simulink model "RL_Satellite_Model"  (R2024b)
settings: Solver=ode4  StartTime=0.0  StopTime=100  FixedStep=0.1  RelTol=1e-3
values from neighbouring files (symbols this model uses):
  debris1_vx = debris1_speed * cos(debris1_angle)    [agent_installation.m]    (also in resetFcn.m = 0.5*vx0 + debris1_speed * cos(dir1))
  debris1_vy = debris1_speed * sin(debris1_angle)    [agent_installation.m]    (also in resetFcn.m = 0.5*vy0 + debris1_speed * sin(dir1))
  debris1_vz = 0    [agent_installation.m]    (also in resetFcn.m = -(500 + rand*1000))
  debris2_vx = debris2_speed * cos(debris2_angle)    [agent_installation.m]    (also in resetFcn.m = 0.5*vx0 + debris2_speed * cos(dir2))
  debris2_vy = debris2_speed * sin(debris2_angle)    [agent_installation.m]    (also in resetFcn.m = 0.5*vy0 + debris2_speed * sin(dir2))
  debris2_vz = 0    [agent_installation.m]    (also in resetFcn.m = +(500 + rand*1000))
  debris3_vx = debris3_speed * cos(debris3_angle)    [agent_installation.m]    (also in resetFcn.m = 0.5*vx0 + debris3_speed * cos(dir3))
  debris3_vy = debris3_speed * sin(debris3_angle)    [agent_installation.m]    (also in resetFcn.m = 0.5*vy0 + debris3_speed * sin(dir3))
  debris3_vz = 0    [agent_installation.m]    (also in resetFcn.m = (rand - 0.5) * 300)
  vx0 = 0    [agent_installation.m]    (also in resetFcn.m = -sqrt(mu/r_target) * sin(sat_angle))
  vy0 = 7546    [agent_installation.m]    (also in resetFcn.m = sqrt(mu/r_target) * cos(sat_angle))
  vz0 = 0    [agent_installation.m]    (also in resetFcn.m)
  x0 = 7e6    (= 7000000)    [agent_installation.m]    (also in resetFcn.m = r_target * cos(sat_angle))
  y0 = 0    [agent_installation.m]    (also in resetFcn.m = r_target * sin(sat_angle))
  z0 = 0    [agent_installation.m]    (also in resetFcn.m = (rand - 0.5) * 2e4)
libraries: simulink x4, rllib x1, vrlib x1
settings Model: PacingRate=20  Creator=Emc  LastModifiedBy=Emc

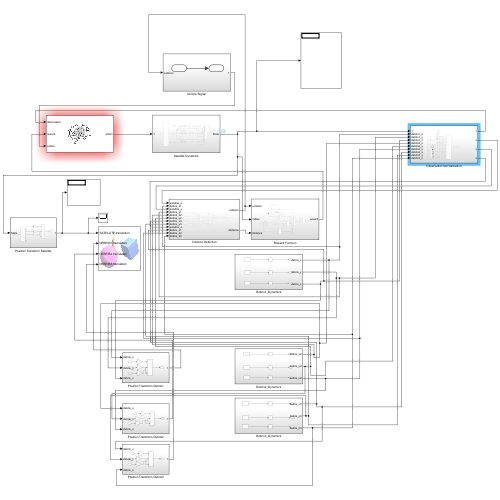
[thumbnail: Simulink's stored preview of the top-level diagram]
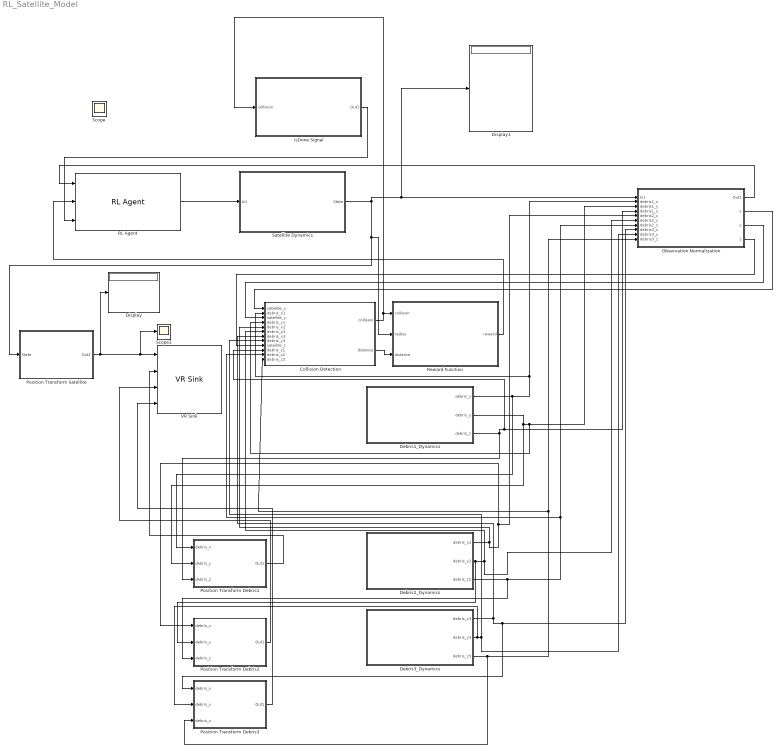
== system RL_Satellite_Model ==
  Collision Detection : Subsystem
  Debris1_Dynamics : Subsystem
  Debris2_Dynamics : Subsystem
  Debris3_Dynamics : Subsystem
  Display : Display
  Display1 : Display
  Observation Normalization : Subsystem
  Position Transform Debris1 : Subsystem
  Position Transform Debris2 : Subsystem
  Position Transform Debris3 : Subsystem
  Position Transform Satellite : Subsystem
  RL Agent : rllib/RL Agent  Agent=agentObj  ExternalActionAsInput=off  ProvideLastAction=off  ProvideCumRwd=off  TreatAsDirectFeedthrough=on  UseStrictObservationDataTypes=off
  Reward Function : Subsystem
  Satellite Dynamics : Subsystem
  Scope1 : Scope
  VR Sink : vrlib/VR Sink  InstantiateOnLoad=on  SampleTime=0.1  ViewEnable=on  RemoteChange=off  RemoteView=off  FieldsWritten=SATELLITE.translation.3.1.1.double#DEBRIS1.translation.3.1.1.double#DEBRIS2.translation.3.1.1.double#DEBRIS3.translation.3.1.1.double  WorldFileName=space_world.wrl  WorldDescription=Satellite Debris Avoidance  AutoView=on  VideoDimensions=[]  AllowVariableSize=off
  isDone Signal : Subsystem
  Scope : Scope
  wires:
  RL Agent/1 -> Satellite Dynamics/1(In1)
  Satellite Dynamics/1(State) -> Reward Function/2(radius), Position Transform Satellite/1(State), Display1/1, Observation Normalization/1(In1)
  Observation Normalization/1(Out1) -> RL Agent/1
  Reward Function/1(reward) -> RL Agent/2
  isDone Signal/1(Out1) -> RL Agent/3
  Debris1_Dynamics/1(debris_x) -> Position Transform Debris1/1(debris_x), Collision Detection/2(debris_x1), Observation Normalization/2(debris1_x)
  Debris1_Dynamics/2(debris_y) -> Position Transform Debris1/2(debris_y), Collision Detection/4(debris_y1), Observation Normalization/3(debris1_y)
  Collision Detection/1(collision) -> isDone Signal/1(collision), Reward Function/1(collision)
  Collision Detection/2(distance) -> Reward Function/3(distance)
  Observation Normalization/2(x) -> Collision Detection/1(satellite_x)
  Observation Normalization/3(y) -> Collision Detection/3(satellite_y)
  Position Transform Satellite/1(Out1) -> VR Sink/1, Scope1/1, Display/1
  Position Transform Debris1/1(Out1) -> VR Sink/2
  Position Transform Debris2/1(Out1) -> VR Sink/3
  Position Transform Debris3/1(Out1) -> VR Sink/4
  Debris2_Dynamics/1(debris_x2) -> Position Transform Debris2/1(debris_x), Observation Normalization/5(debris2_x), Collision Detection/5(debris_x2)
  Debris2_Dynamics/2(debris_y2) -> Position Transform Debris2/2(debris_y), Observation Normalization/6(debris2_y), Collision Detection/6(debris_y2)
  Debris3_Dynamics/1(debris_x3) -> Position Transform Debris3/1(debris_x), Observation Normalization/8(debris3_x), Collision Detection/7(debris_x3)
  Debris3_Dynamics/2(debris_y3) -> Position Transform Debris3/2(debris_y), Observation Normalization/9(debris3_y), Collision Detection/8(debris_y3)
  Debris1_Dynamics/3(debris_z) -> Position Transform Debris1/3(debris_z), Observation Normalization/4(debris1_z), Collision Detection/10(debris_z1)
  Debris2_Dynamics/3(debris_z2) -> Position Transform Debris2/3(debris_z), Collision Detection/11(debris_z2), Observation Normalization/7(debris2_z)
  Debris3_Dynamics/3(debris_z3) -> Position Transform Debris3/3(debris_z), Collision Detection/12(debris_z3), Observation Normalization/10(debris3_z)
  Observation Normalization/4(z) -> Collision Detection/9(satellite_z)

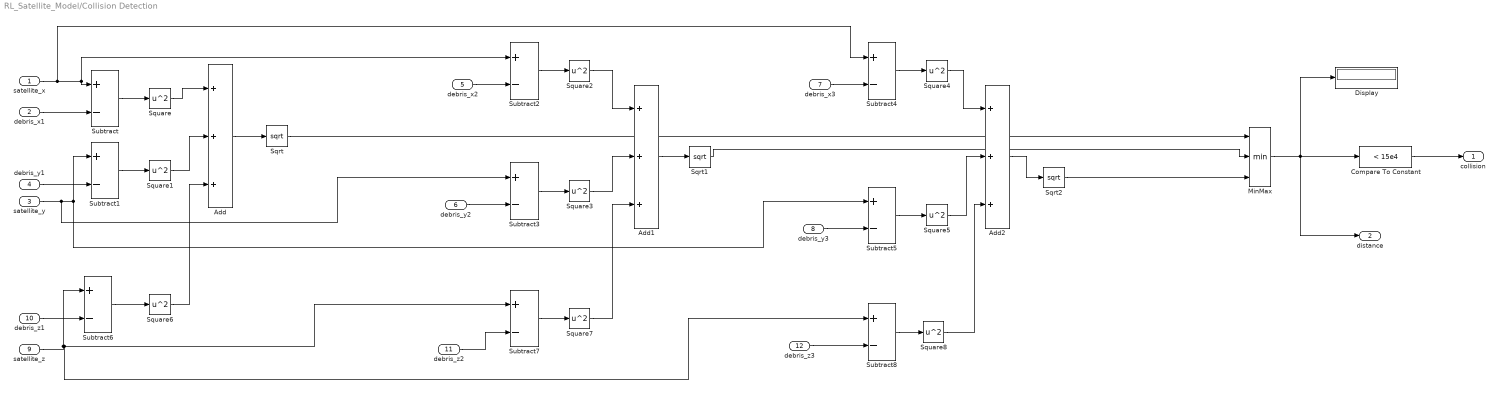
== system RL_Satellite_Model/Collision Detection ==
  satellite_x : Inport
  debris_x1 : Inport  Port=2
  satellite_y : Inport  Port=3
  debris_y1 : Inport  Port=4
  debris_x2 : Inport  Port=5
  debris_y2 : Inport  Port=6
  debris_x3 : Inport  Port=7
  debris_y3 : Inport  Port=8
  satellite_z : Inport  Port=9
  debris_z1 : Inport  Port=10
  debris_z2 : Inport  Port=11
  debris_z3 : Inport  Port=12
  Add : Sum  Inputs=+++
  Add1 : Sum  Inputs=+++
  Add2 : Sum  Inputs=+++
  Compare To Constant : simulink/Logic and Bit Operations/Compare To Constant  relop=<  const=15e4  OutDataTypeStr=boolean
  Display : Display
  MinMax : MinMax  Inputs=3
  Sqrt : Sqrt
  Sqrt1 : Sqrt
  Sqrt2 : Sqrt
  Square{,1..8} (9 alike) : Math  Operator=square
  Subtract{,1..8} (9 alike) : Sum  Inputs=+-
  collision : Outport
  distance : Outport  Port=2
  wires:
  debris_x1/1 -> Subtract/2
  Subtract/1 -> Square/1
  debris_y1/1 -> Subtract1/2
  Subtract1/1 -> Square1/1
  Square/1 -> Add/1
  Square1/1 -> Add/2
  Add/1 -> Sqrt/1
  Sqrt/1 -> MinMax/1
  Add1/1 -> Sqrt1/1
  Subtract2/1 -> Square2/1
  debris_x2/1 -> Subtract2/2
  Square3/1 -> Add1/2
  satellite_x/1 -> Subtract4/1, Subtract2/1, Subtract/1
  debris_y2/1 -> Subtract3/2
  satellite_y/1 -> Subtract3/1, Subtract5/1, Subtract1/1
  Square2/1 -> Add1/1
  Subtract3/1 -> Square3/1
  Subtract5/1 -> Square5/1
  Square4/1 -> Add2/1
  Square5/1 -> Add2/2
  Subtract4/1 -> Square4/1
  Add2/1 -> Sqrt2/1
  debris_x3/1 -> Subtract4/2
  debris_y3/1 -> Subtract5/2
  Sqrt1/1 -> MinMax/2
  Sqrt2/1 -> MinMax/3
  MinMax/1 -> Compare To Constant/1, distance/1, Display/1
  Compare To Constant/1 -> collision/1
  satellite_z/1 -> Subtract8/1, Subtract7/1, Subtract6/1
  debris_z1/1 -> Subtract6/2
  Subtract6/1 -> Square6/1
  Square6/1 -> Add/3
  debris_z2/1 -> Subtract7/2
  Subtract7/1 -> Square7/1
  Square7/1 -> Add1/3
  debris_z3/1 -> Subtract8/2
  Subtract8/1 -> Square8/1
  Square8/1 -> Add2/3

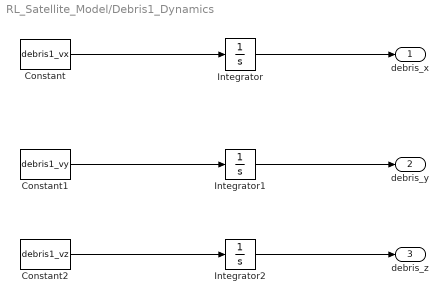
== system RL_Satellite_Model/Debris1_Dynamics ==
  Constant : Constant  Value=debris1_vx
  Constant1 : Constant  Value=debris1_vy
  Constant2 : Constant  Value=debris1_vz
  Integrator : Integrator  InitialCondition=4211716.8255
  Integrator1 : Integrator  InitialCondition=-5267255.8785
  Integrator2 : Integrator  InitialCondition=-7549.9128
  debris_x : Outport
  debris_y : Outport  Port=2
  debris_z : Outport  Port=3
  wires:
  Integrator/1 -> debris_x/1
  Integrator1/1 -> debris_y/1
  Constant/1 -> Integrator/1
  Constant1/1 -> Integrator1/1
  Integrator2/1 -> debris_z/1
  Constant2/1 -> Integrator2/1

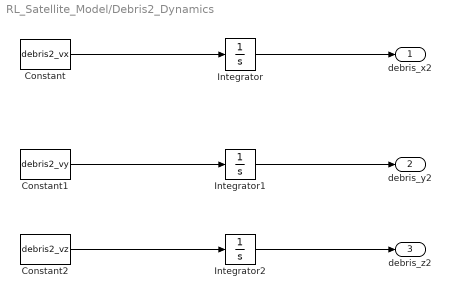
== system RL_Satellite_Model/Debris2_Dynamics ==
  Constant : Constant  Value=debris2_vx
  Constant1 : Constant  Value=debris2_vy
  Constant2 : Constant  Value=debris2_vz
  Integrator : Integrator  InitialCondition=4531915.4516
  Integrator1 : Integrator  InitialCondition=-5612092.005
  Integrator2 : Integrator  InitialCondition=-1728.006
  debris_x2 : Outport
  debris_y2 : Outport  Port=2
  debris_z2 : Outport  Port=3
  wires:
  Integrator/1 -> debris_x2/1
  Integrator1/1 -> debris_y2/1
  Constant/1 -> Integrator/1
  Constant1/1 -> Integrator1/1
  Integrator2/1 -> debris_z2/1
  Constant2/1 -> Integrator2/1

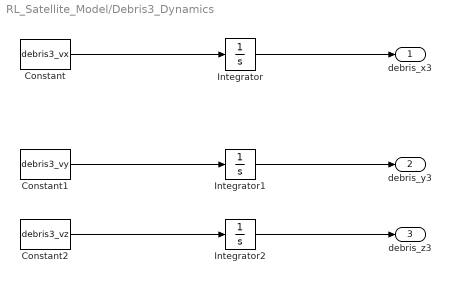
== system RL_Satellite_Model/Debris3_Dynamics ==
  Constant : Constant  Value=debris3_vx
  Constant1 : Constant  Value=debris3_vy
  Constant2 : Constant  Value=debris3_vz
  Integrator : Integrator  InitialCondition=4454904.9368
  Integrator1 : Integrator  InitialCondition=-5298697.3695
  Integrator2 : Integrator  InitialCondition=8872.5823
  debris_x3 : Outport
  debris_y3 : Outport  Port=2
  debris_z3 : Outport  Port=3
  wires:
  Integrator/1 -> debris_x3/1
  Integrator1/1 -> debris_y3/1
  Constant/1 -> Integrator/1
  Constant1/1 -> Integrator1/1
  Constant2/1 -> Integrator2/1
  Integrator2/1 -> debris_z3/1

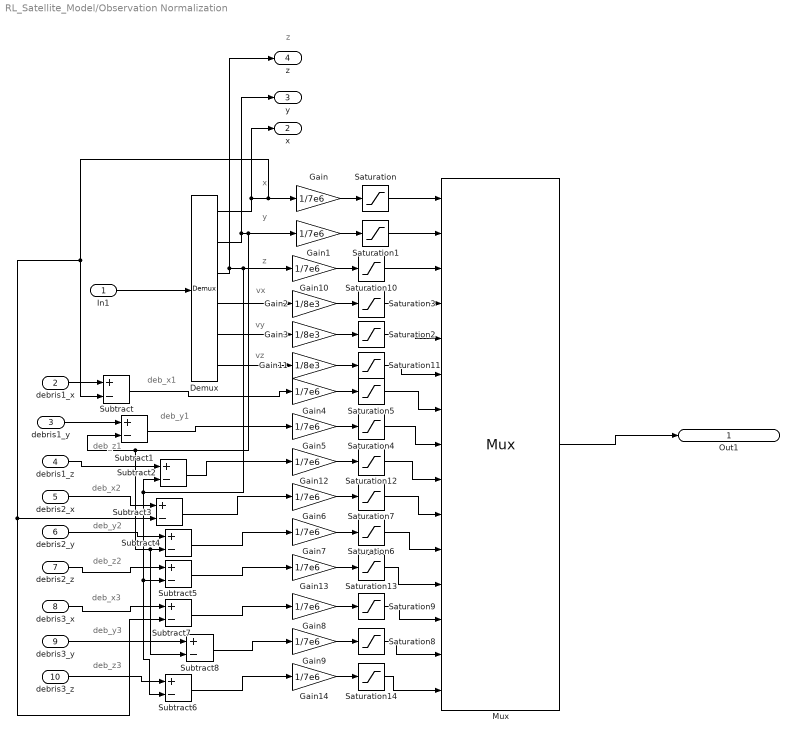
== system RL_Satellite_Model/Observation Normalization ==
  note: z
  note: deb_x1
  note: y
  note: x
  note: deb_y1
  note: deb_x2
  note: deb_y2
  note: deb_x3
  note: deb_y3
  note: vy
  note: vx
  note: z
  note: vz
  note: deb_z1
  note: deb_z2
  note: deb_z3
  In1 : Inport
  debris1_x : Inport  Port=2
  debris1_y : Inport  Port=3
  debris1_z : Inport  Port=4
  debris2_x : Inport  Port=5
  debris2_y : Inport  Port=6
  debris2_z : Inport  Port=7
  debris3_x : Inport  Port=8
  debris3_y : Inport  Port=9
  debris3_z : Inport  Port=10
  Demux : Demux  Outputs=6
      settings: DisplayOption=none
  Gain{,1,4..10,12..14} (12 alike) : Gain  Gain=1/7e6
  Gain11 : Gain  Gain=1/8e3
  Gain2 : Gain  Gain=1/8e3
  Gain3 : Gain  Gain=1/8e3
  Mux : Mux  Inputs=15
      settings: DisplayOption=signals
  Saturation{,1..14} (15 alike) : Saturate  UpperLimit=2  LowerLimit=-2
  Subtract{,1..8} (9 alike) : Sum  Inputs=+-
  Out1 : Outport
  x : Outport  Port=2
  y : Outport  Port=3
  z : Outport  Port=4
  wires:
  Demux/1 -> x/1, Subtract/2, Subtract7/2, Subtract3/2, Gain/1
  Demux/2 -> Gain1/1, Subtract1/2, Subtract8/2, Subtract4/2, y/1
  Gain/1 -> Saturation/1
  Gain1/1 -> Saturation1/1
  Saturation/1 -> Mux/1
  Saturation1/1 -> Mux/2
  Gain5/1 -> Saturation4/1
  Gain4/1 -> Saturation5/1
  In1/1 -> Demux/1
  Gain7/1 -> Saturation6/1
  Gain6/1 -> Saturation7/1
  Gain9/1 -> Saturation8/1
  Gain8/1 -> Saturation9/1
  Gain2/1 -> Saturation3/1
  Demux/5 -> Gain3/1
  Demux/4 -> Gain2/1
  Gain3/1 -> Saturation2/1
  Demux/3 -> z/1, Subtract6/2, Subtract5/2, Subtract2/2, Gain10/1
  Gain10/1 -> Saturation10/1
  Saturation10/1 -> Mux/3
  Saturation3/1 -> Mux/4
  Saturation2/1 -> Mux/5
  Mux/1 -> Out1/1
  Demux/6 -> Gain11/1
  Saturation11/1 -> Mux/6
  Gain11/1 -> Saturation11/1
  Saturation5/1 -> Mux/7
  Saturation4/1 -> Mux/8
  Gain12/1 -> Saturation12/1
  Saturation12/1 -> Mux/9
  Gain13/1 -> Saturation13/1
  Saturation7/1 -> Mux/10
  Saturation6/1 -> Mux/11
  Saturation13/1 -> Mux/12
  Gain14/1 -> Saturation14/1
  Saturation9/1 -> Mux/13
  Saturation8/1 -> Mux/14
  Saturation14/1 -> Mux/15
  debris1_x/1 -> Subtract/1
  Subtract/1 -> Gain4/1
  debris1_y/1 -> Subtract1/1
  debris1_z/1 -> Subtract2/1
  Subtract1/1 -> Gain5/1
  Subtract2/1 -> Gain12/1
  debris2_x/1 -> Subtract3/1
  Subtract3/1 -> Gain6/1
  debris2_y/1 -> Subtract4/1
  Subtract4/1 -> Gain7/1
  debris2_z/1 -> Subtract5/1
  debris3_z/1 -> Subtract6/1
  Subtract5/1 -> Gain13/1
  debris3_x/1 -> Subtract7/1
  Subtract7/1 -> Gain8/1
  Subtract6/1 -> Gain14/1
  debris3_y/1 -> Subtract8/1
  Subtract8/1 -> Gain9/1

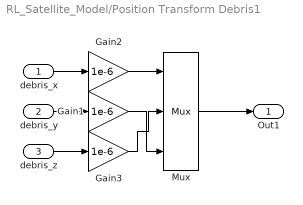
== system RL_Satellite_Model/Position Transform Debris1 ==
  debris_x : Inport
  debris_y : Inport  Port=2
  debris_z : Inport  Port=3
  Gain1 : Gain  Gain=1e-6
  Gain2 : Gain  Gain=1e-6
  Gain3 : Gain  Gain=1e-6
  Mux : Mux  Inputs=3
      settings: DisplayOption=signals
  Out1 : Outport
  wires:
  Gain2/1 -> Mux/1
  Mux/1 -> Out1/1
  debris_x/1 -> Gain2/1
  debris_z/1 -> Gain3/1
  debris_y/1 -> Gain1/1
  Gain1/1 -> Mux/3
  Gain3/1 -> Mux/2

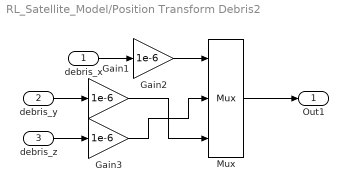
== system RL_Satellite_Model/Position Transform Debris2 ==
  debris_x : Inport
  debris_y : Inport  Port=2
  debris_z : Inport  Port=3
  Gain1 : Gain  Gain=1e-6
  Gain2 : Gain  Gain=1e-6
  Gain3 : Gain  Gain=1e-6
  Mux : Mux  Inputs=3
      settings: DisplayOption=signals
  Out1 : Outport
  wires:
  Mux/1 -> Out1/1
  debris_y/1 -> Gain1/1
  debris_x/1 -> Gain2/1
  Gain2/1 -> Mux/1
  debris_z/1 -> Gain3/1
  Gain1/1 -> Mux/3
  Gain3/1 -> Mux/2

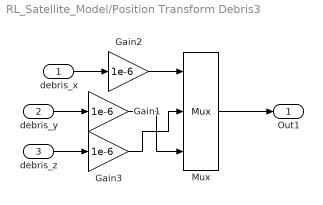
== system RL_Satellite_Model/Position Transform Debris3 ==
  debris_x : Inport
  debris_y : Inport  Port=2
  debris_z : Inport  Port=3
  Gain1 : Gain  Gain=1e-6
  Gain2 : Gain  Gain=1e-6
  Gain3 : Gain  Gain=1e-6
  Mux : Mux  Inputs=3
      settings: DisplayOption=signals
  Out1 : Outport
  wires:
  Mux/1 -> Out1/1
  debris_y/1 -> Gain1/1
  debris_x/1 -> Gain2/1
  Gain2/1 -> Mux/1
  debris_z/1 -> Gain3/1
  Gain1/1 -> Mux/3
  Gain3/1 -> Mux/2

== system RL_Satellite_Model/Position Transform Satellite ==
  note: x
  note: y
  note: z
  State : Inport
  Demux : Demux  Outputs=6
      settings: DisplayOption=none
  Gain : Gain  Gain=1e-6
  Gain1 : Gain  Gain=1e-6
  Gain2 : Gain  Gain=1e-6
  Mux : Mux  Inputs=3
      settings: DisplayOption=signals
  Out1 : Outport
  wires:
  State/1 -> Demux/1
  Mux/1 -> Out1/1
  Gain/1 -> Mux/1
  Demux/1 -> Gain/1
  Demux/2 -> Gain1/1
  Demux/3 -> Gain2/1
  Gain1/1 -> Mux/3
  Gain2/1 -> Mux/2

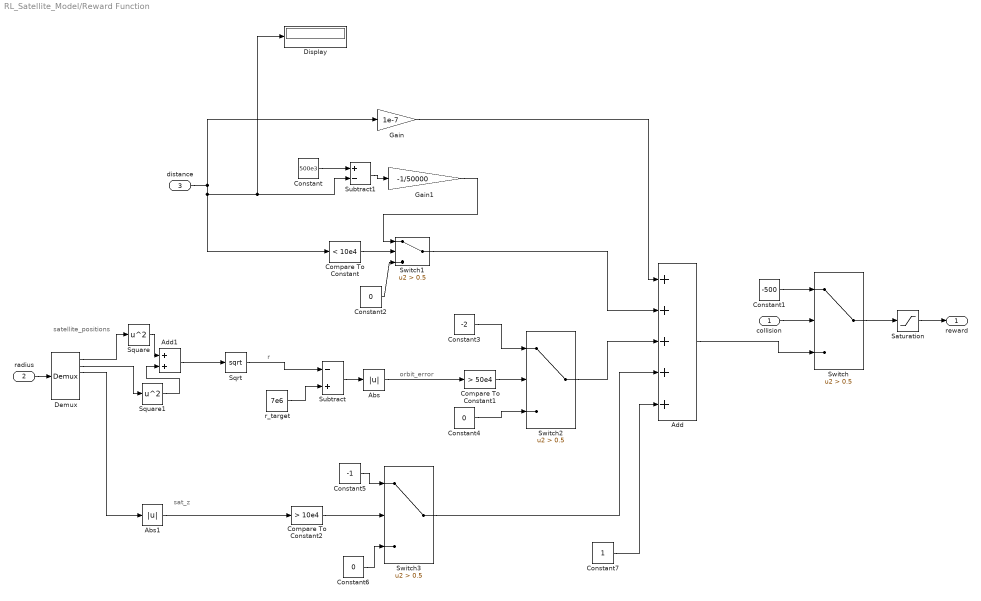
== system RL_Satellite_Model/Reward Function ==
  note: sat_z
  note: orbit_error
  note: r
  note: satellite_positions
  collision : Inport
  radius : Inport  Port=2
  distance : Inport  Port=3
  Abs : Abs  SaturateOnIntegerOverflow=off
  Abs1 : Abs  SaturateOnIntegerOverflow=off
  Add : Sum  Inputs=+++++
  Add1 : Sum
  Compare To Constant : simulink/Logic and Bit Operations/Compare To Constant  relop=<  const=10e4  OutDataTypeStr=boolean
  Compare To Constant1 : simulink/Logic and Bit Operations/Compare To Constant  relop=>  const=50e4  OutDataTypeStr=boolean
  Compare To Constant2 : simulink/Logic and Bit Operations/Compare To Constant  relop=>  const=10e4  OutDataTypeStr=boolean
  Constant : Constant  Value=500e3
  Constant1 : Constant  Value=-500
  Constant2 : Constant  Value=0
  Constant3 : Constant  Value=-2
  Constant4 : Constant  Value=0
  Constant5 : Constant  Value=-1
  Constant6 : Constant  Value=0
  Constant7 : Constant
  Demux : Demux  Outputs=6
      settings: DisplayOption=none
  Display : Display
  Gain : Gain  Gain=1e-7
  Gain1 : Gain  Gain=-1/50000
  Saturation : Saturate  UpperLimit=100  LowerLimit=-100
  Sqrt : Sqrt
  Square : Math  Operator=square
  Square1 : Math  Operator=square
  Subtract : Sum  Inputs=-+
  Subtract1 : Sum  Inputs=+-
  Switch{,1..3} (4 alike) : Switch  Criteria=u2 > Threshold  Threshold=0.5  SaturateOnIntegerOverflow=off  InputSameDT=off
  r_target : Constant  Value=7e6
  reward : Outport
  wires:
  distance/1 -> Display/1, Subtract1/2, Compare To Constant/1, Gain/1
  collision/1 -> Switch/2
  Constant1/1 -> Switch/1
  Switch/1 -> Saturation/1
  Saturation/1 -> reward/1
  Compare To Constant/1 -> Switch1/2
  Gain1/1 -> Switch1/1
  Constant2/1 -> Switch1/3
  Switch1/1 -> Add/2
  Gain/1 -> Add/1
  Add/1 -> Switch/3
  radius/1 -> Demux/1
  Demux/1 -> Square/1
  Demux/2 -> Square1/1
  Add1/1 -> Sqrt/1
  Sqrt/1 -> Subtract/1
  r_target/1 -> Subtract/2
  Subtract/1 -> Abs/1
  Abs/1 -> Compare To Constant1/1
  Constant3/1 -> Switch2/1
  Constant4/1 -> Switch2/3
  Switch2/1 -> Add/3
  Abs1/1 -> Compare To Constant2/1
  Compare To Constant2/1 -> Switch3/2
  Constant5/1 -> Switch3/1
  Constant6/1 -> Switch3/3
  Switch3/1 -> Add/4
  Compare To Constant1/1 -> Switch2/2
  Square/1 -> Add1/1
  Square1/1 -> Add1/2
  Demux/3 -> Abs1/1
  Constant/1 -> Subtract1/1
  Subtract1/1 -> Gain1/1
  Constant7/1 -> Add/5

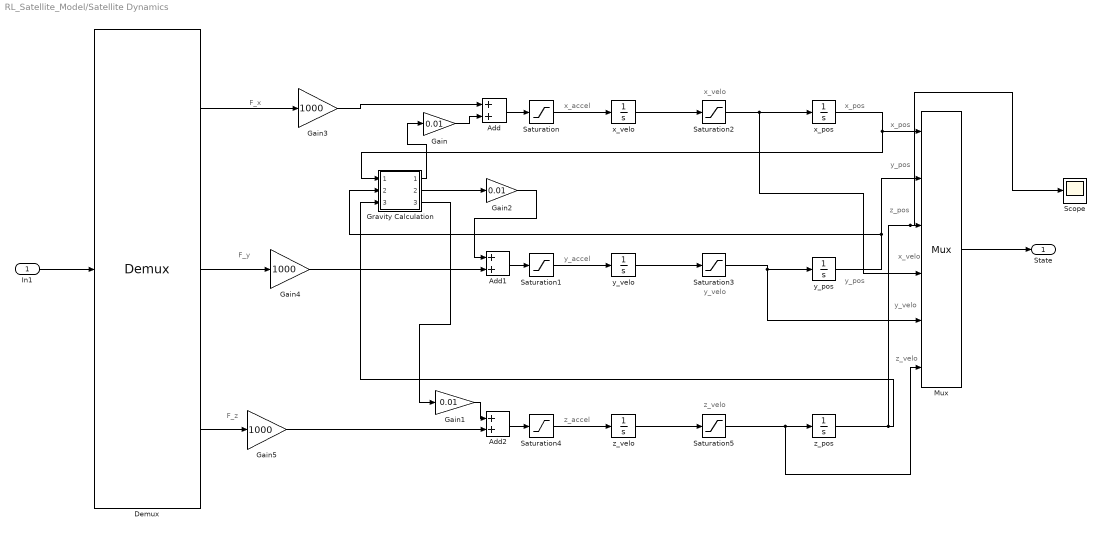
== system RL_Satellite_Model/Satellite Dynamics ==
  note: z_velo
  note: x_pos
  note: x_accel
  note: F_y
  note: F_x
  note: y_accel
  note: x_velo
  note: y_velo
  note: y_pos
  note: x_pos
  note: y_pos
  note: z_pos
  note: x_velo
  note: F_z
  note: z_velo
  note: z_accel
  note: y_velo
  In1 : Inport
  Add : Sum
  Add1 : Sum
  Add2 : Sum
  Demux : Demux  Outputs=3
      settings: DisplayOption=none
  Gain : Gain  Gain=0.01
  Gain1 : Gain  Gain=0.01
  Gain2 : Gain  Gain=0.01
  Gain3 : Gain  Gain=1000
  Gain4 : Gain  Gain=1000
  Gain5 : Gain  Gain=1000
  Gravity Calculation : Subsystem
  Mux : Mux  Inputs=6
      settings: DisplayOption=signals
  Saturation : Saturate  UpperLimit=100  LowerLimit=-100
  Saturation1 : Saturate  UpperLimit=100  LowerLimit=-100
  Saturation2 : Saturate  UpperLimit=50e3  LowerLimit=-50e3
  Saturation3 : Saturate  UpperLimit=50e3  LowerLimit=-50e3
  Saturation4 : Saturate  UpperLimit=100  LowerLimit=-100
  Saturation5 : Saturate  UpperLimit=50e3  LowerLimit=-50e3
  Scope : Scope
  x_pos : Integrator  InitialCondition=x0
  x_velo : Integrator  InitialCondition=vx0
  y_pos : Integrator  InitialCondition=y0
  y_velo : Integrator  InitialCondition=vy0
  z_pos : Integrator  InitialCondition=z0
  z_velo : Integrator  InitialCondition=vz0
  State : Outport
  wires:
  In1/1 -> Demux/1
  Demux/2 -> Gain4/1
  Demux/1 -> Gain3/1
  Gain3/1 -> Add/1
  Saturation/1 -> x_velo/1
  Gain4/1 -> Add1/2
  Saturation1/1 -> y_velo/1
  y_velo/1 -> Saturation3/1
  x_velo/1 -> Saturation2/1
  y_pos/1 -> Mux/2, Gravity Calculation/2(y_pos)
  x_pos/1 -> Gravity Calculation/1(x_pos), Mux/1
  Gravity Calculation/1(Out1) -> Gain/1
  Add/1 -> Saturation/1
  Add1/1 -> Saturation1/1
  Mux/1 -> State/1
  Saturation2/1 -> Mux/4, x_pos/1
  Saturation3/1 -> Mux/5, y_pos/1
  Gain5/1 -> Add2/2
  Add2/1 -> Saturation4/1
  Saturation4/1 -> z_velo/1
  z_velo/1 -> Saturation5/1
  Saturation5/1 -> z_pos/1, Mux/6
  Demux/3 -> Gain5/1
  z_pos/1 -> Scope/1, Mux/3, Gravity Calculation/3(z_pos)
  Gain/1 -> Add/2
  Gravity Calculation/2(Out2) -> Gain2/1
  Gain2/1 -> Add1/1
  Gravity Calculation/3(Out3) -> Gain1/1
  Gain1/1 -> Add2/1

== system RL_Satellite_Model/isDone Signal ==
  collision : Inport
  Out1 : Outport
  wires:
  collision/1 -> Out1/1

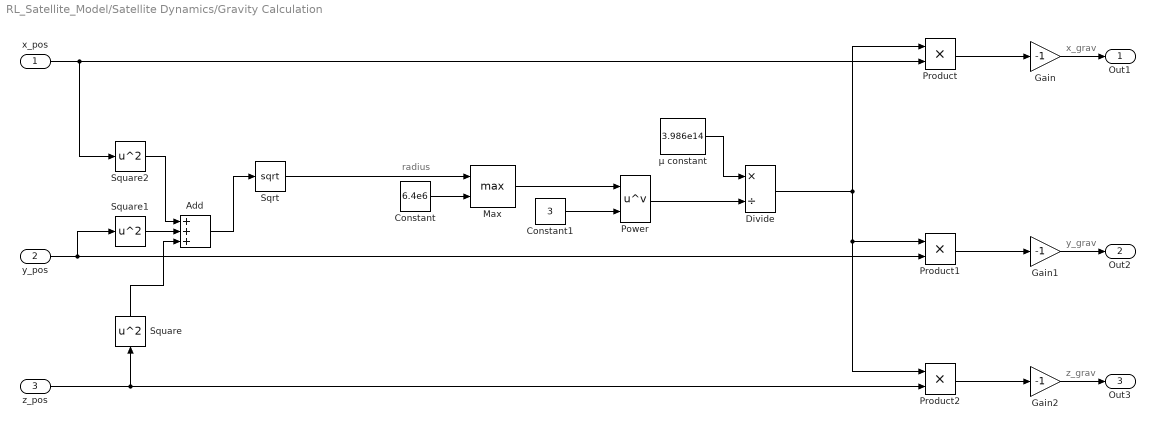
== system RL_Satellite_Model/Satellite Dynamics/Gravity Calculation ==
  note: x_grav
  note: radius
  note: y_grav
  note: z_grav
  x_pos : Inport
  y_pos : Inport  Port=2
  z_pos : Inport  Port=3
  " μ constant" : Constant  Value=3.986e14
  Add : Sum  Inputs=+++
  Constant : Constant  Value=6.4e6
  Constant1 : Constant  Value=3
  Divide : Product  Inputs=*/
  Gain : Gain  Gain=-1
  Gain1 : Gain  Gain=-1
  Gain2 : Gain  Gain=-1
  Max : MinMax  Function=max  Inputs=2
  Power : Math  Operator=pow
  Product : Product
  Product1 : Product
  Product2 : Product
  Sqrt : Sqrt
  Square : Math  Operator=square
  Square1 : Math  Operator=square
  Square2 : Math  Operator=square
  Out1 : Outport
  Out2 : Outport  Port=2
  Out3 : Outport  Port=3
  wires:
  x_pos/1 -> Product/2, Square2/1
  y_pos/1 -> Square1/1, Product1/2
  Sqrt/1 -> Max/1
  Constant/1 -> Max/2
  Max/1 -> Power/1
  Constant1/1 -> Power/2
  " μ constant"/1 -> Divide/1
  Power/1 -> Divide/2
  Product1/1 -> Gain1/1
  Divide/1 -> Product/1, Product2/1, Product1/1
  Product/1 -> Gain/1
  Gain1/1 -> Out2/1
  Gain/1 -> Out1/1
  Product2/1 -> Gain2/1
  Gain2/1 -> Out3/1
  z_pos/1 -> Product2/2, Square/1
  Square2/1 -> Add/1
  Square1/1 -> Add/2
  Square/1 -> Add/3
  Add/1 -> Sqrt/1
